simulink model "pi_SS_H2DF_2024a_GRU"  (R2024a)
settings: Solver=FixedStepAuto  StartTime=0.0  StopTime=inf  FixedStep=0.001  RelTol=1e-3  EnableMultiTasking=on
values from neighbouring files (symbols this model uses):
  C2C_NMPC = init_C2C_NMPC_H2DF(C2C_NMPC.expdata)    [run_SS_H2DF_control.m]
libraries: matrix_library x3, raspberrypiNetworklib x1
(part 3 of 3)

== system pi_SS_H2DF_2024a_GRU/main_C2C/post_processing/Subsystem1/Subsystem ==
  In1 : Inport
  In2 : Inport  Port=2
  In3 : Inport  Port=3
  In4 : Inport  Port=4
  " denormalizing reference1" : Subsystem
  " denormalizing reference2" : Subsystem
  " denormalizing reference3" : Subsystem
  " denormalizing reference4" : Subsystem
  Demux{,1..3} (4 alike) : Demux
  Mux{,1..3} (4 alike) : Mux
  Node_0 : Outport
  Node_1 : Outport  Port=2
  Node_2 : Outport  Port=3
  Node_3 : Outport  Port=4
  wires:
  Demux/1 -> " denormalizing reference1"/1(IMEP_norm)
  Demux/2 -> " denormalizing reference1"/2(NOX_norm)
  Demux/3 -> " denormalizing reference1"/3(soot_norm)
  Demux/4 -> " denormalizing reference1"/4(MPRR_norm)
  In1/1 -> Demux/1
  " denormalizing reference1"/1(IMEP) -> Mux/1
  " denormalizing reference1"/2(NOX) -> Mux/2
  " denormalizing reference1"/3(soot) -> Mux/3
  " denormalizing reference1"/4(MPRR) -> Mux/4
  " denormalizing reference2"/3(soot) -> Mux1/3
  Demux1/3 -> " denormalizing reference2"/3(soot_norm)
  In2/1 -> Demux1/1
  " denormalizing reference2"/2(NOX) -> Mux1/2
  " denormalizing reference2"/1(IMEP) -> Mux1/1
  Demux1/1 -> " denormalizing reference2"/1(IMEP_norm)
  Demux1/4 -> " denormalizing reference2"/4(MPRR_norm)
  Demux1/2 -> " denormalizing reference2"/2(NOX_norm)
  " denormalizing reference2"/4(MPRR) -> Mux1/4
  " denormalizing reference3"/3(soot) -> Mux2/3
  Demux2/3 -> " denormalizing reference3"/3(soot_norm)
  In3/1 -> Demux2/1
  " denormalizing reference3"/2(NOX) -> Mux2/2
  " denormalizing reference3"/1(IMEP) -> Mux2/1
  Demux2/1 -> " denormalizing reference3"/1(IMEP_norm)
  Demux2/4 -> " denormalizing reference3"/4(MPRR_norm)
  Demux2/2 -> " denormalizing reference3"/2(NOX_norm)
  " denormalizing reference3"/4(MPRR) -> Mux2/4
  " denormalizing reference4"/3(soot) -> Mux3/3
  Demux3/3 -> " denormalizing reference4"/3(soot_norm)
  In4/1 -> Demux3/1
  " denormalizing reference4"/2(NOX) -> Mux3/2
  " denormalizing reference4"/1(IMEP) -> Mux3/1
  Demux3/1 -> " denormalizing reference4"/1(IMEP_norm)
  Demux3/4 -> " denormalizing reference4"/4(MPRR_norm)
  Demux3/2 -> " denormalizing reference4"/2(NOX_norm)
  " denormalizing reference4"/4(MPRR) -> Mux3/4
  Mux/1 -> Node_0/1
  Mux1/1 -> Node_1/1
  Mux2/1 -> Node_2/1
  Mux3/1 -> Node_3/1

== system pi_SS_H2DF_2024a_GRU/main_C2C/post_processing/Subsystem1/Subsystem/ denormalizing reference1 ==
  IMEP_norm : Inport
  NOX_norm : Inport  Port=2
  soot_norm : Inport  Port=3
  MPRR_norm : Inport  Port=4
  Constant : Constant  Value=C2C_NMPC.Normalization.outputs.mean(1)
  Constant1 : Constant  Value=C2C_NMPC.Normalization.outputs.mean(2)
  Constant2 : Constant  Value=C2C_NMPC.Normalization.outputs.mean(3)
  Constant3 : Constant  Value=C2C_NMPC.Normalization.outputs.mean(4)
  Gain : Gain  Gain=C2C_NMPC.Normalization.outputs.std(1)
  Gain1 : Gain  Gain=C2C_NMPC.Normalization.outputs.std(2)
  Gain2 : Gain  Gain=C2C_NMPC.Normalization.outputs.std(3)
  Gain3 : Gain  Gain=C2C_NMPC.Normalization.outputs.std(4)
  Sum{1..3,5} (4 alike) : Sum  Inputs=|++
  IMEP : Outport
  NOX : Outport  Port=2
  soot : Outport  Port=3
  MPRR : Outport  Port=4
  wires:
  Gain/1 -> Sum5/1
  IMEP_norm/1 -> Gain/1
  Constant/1 -> Sum5/2
  Sum5/1 -> IMEP/1
  Gain1/1 -> Sum1/1
  Constant1/1 -> Sum1/2
  NOX_norm/1 -> Gain1/1
  Sum1/1 -> NOX/1
  Gain2/1 -> Sum2/1
  Constant2/1 -> Sum2/2
  soot_norm/1 -> Gain2/1
  Sum2/1 -> soot/1
  Gain3/1 -> Sum3/1
  Constant3/1 -> Sum3/2
  MPRR_norm/1 -> Gain3/1
  Sum3/1 -> MPRR/1

== system pi_SS_H2DF_2024a_GRU/main_C2C/post_processing/Subsystem1/Subsystem/ denormalizing reference2 ==
  IMEP_norm : Inport
  NOX_norm : Inport  Port=2
  soot_norm : Inport  Port=3
  MPRR_norm : Inport  Port=4
  Constant : Constant  Value=C2C_NMPC.Normalization.outputs.mean(1)
  Constant1 : Constant  Value=C2C_NMPC.Normalization.outputs.mean(2)
  Constant2 : Constant  Value=C2C_NMPC.Normalization.outputs.mean(3)
  Constant3 : Constant  Value=C2C_NMPC.Normalization.outputs.mean(4)
  Gain : Gain  Gain=C2C_NMPC.Normalization.outputs.std(1)
  Gain1 : Gain  Gain=C2C_NMPC.Normalization.outputs.std(2)
  Gain2 : Gain  Gain=C2C_NMPC.Normalization.outputs.std(3)
  Gain3 : Gain  Gain=C2C_NMPC.Normalization.outputs.std(4)
  Sum{1..3,5} (4 alike) : Sum  Inputs=|++
  IMEP : Outport
  NOX : Outport  Port=2
  soot : Outport  Port=3
  MPRR : Outport  Port=4
  wires:
  Gain/1 -> Sum5/1
  IMEP_norm/1 -> Gain/1
  Constant/1 -> Sum5/2
  Sum5/1 -> IMEP/1
  Gain1/1 -> Sum1/1
  Constant1/1 -> Sum1/2
  NOX_norm/1 -> Gain1/1
  Sum1/1 -> NOX/1
  Gain2/1 -> Sum2/1
  Constant2/1 -> Sum2/2
  soot_norm/1 -> Gain2/1
  Sum2/1 -> soot/1
  Gain3/1 -> Sum3/1
  Constant3/1 -> Sum3/2
  MPRR_norm/1 -> Gain3/1
  Sum3/1 -> MPRR/1

== system pi_SS_H2DF_2024a_GRU/main_C2C/post_processing/Subsystem1/Subsystem/ denormalizing reference3 ==
  IMEP_norm : Inport
  NOX_norm : Inport  Port=2
  soot_norm : Inport  Port=3
  MPRR_norm : Inport  Port=4
  Constant : Constant  Value=C2C_NMPC.Normalization.outputs.mean(1)
  Constant1 : Constant  Value=C2C_NMPC.Normalization.outputs.mean(2)
  Constant2 : Constant  Value=C2C_NMPC.Normalization.outputs.mean(3)
  Constant3 : Constant  Value=C2C_NMPC.Normalization.outputs.mean(4)
  Gain : Gain  Gain=C2C_NMPC.Normalization.outputs.std(1)
  Gain1 : Gain  Gain=C2C_NMPC.Normalization.outputs.std(2)
  Gain2 : Gain  Gain=C2C_NMPC.Normalization.outputs.std(3)
  Gain3 : Gain  Gain=C2C_NMPC.Normalization.outputs.std(4)
  Sum{1..3,5} (4 alike) : Sum  Inputs=|++
  IMEP : Outport
  NOX : Outport  Port=2
  soot : Outport  Port=3
  MPRR : Outport  Port=4
  wires:
  Gain/1 -> Sum5/1
  IMEP_norm/1 -> Gain/1
  Constant/1 -> Sum5/2
  Sum5/1 -> IMEP/1
  Gain1/1 -> Sum1/1
  Constant1/1 -> Sum1/2
  NOX_norm/1 -> Gain1/1
  Sum1/1 -> NOX/1
  Gain2/1 -> Sum2/1
  Constant2/1 -> Sum2/2
  soot_norm/1 -> Gain2/1
  Sum2/1 -> soot/1
  Gain3/1 -> Sum3/1
  Constant3/1 -> Sum3/2
  MPRR_norm/1 -> Gain3/1
  Sum3/1 -> MPRR/1

== system pi_SS_H2DF_2024a_GRU/main_C2C/post_processing/Subsystem1/Subsystem/ denormalizing reference4 ==
  IMEP_norm : Inport
  NOX_norm : Inport  Port=2
  soot_norm : Inport  Port=3
  MPRR_norm : Inport  Port=4
  Constant : Constant  Value=C2C_NMPC.Normalization.outputs.mean(1)
  Constant1 : Constant  Value=C2C_NMPC.Normalization.outputs.mean(2)
  Constant2 : Constant  Value=C2C_NMPC.Normalization.outputs.mean(3)
  Constant3 : Constant  Value=C2C_NMPC.Normalization.outputs.mean(4)
  Gain : Gain  Gain=C2C_NMPC.Normalization.outputs.std(1)
  Gain1 : Gain  Gain=C2C_NMPC.Normalization.outputs.std(2)
  Gain2 : Gain  Gain=C2C_NMPC.Normalization.outputs.std(3)
  Gain3 : Gain  Gain=C2C_NMPC.Normalization.outputs.std(4)
  Sum{1..3,5} (4 alike) : Sum  Inputs=|++
  IMEP : Outport
  NOX : Outport  Port=2
  soot : Outport  Port=3
  MPRR : Outport  Port=4
  wires:
  Gain/1 -> Sum5/1
  IMEP_norm/1 -> Gain/1
  Constant/1 -> Sum5/2
  Sum5/1 -> IMEP/1
  Gain1/1 -> Sum1/1
  Constant1/1 -> Sum1/2
  NOX_norm/1 -> Gain1/1
  Sum1/1 -> NOX/1
  Gain2/1 -> Sum2/1
  Constant2/1 -> Sum2/2
  soot_norm/1 -> Gain2/1
  Sum2/1 -> soot/1
  Gain3/1 -> Sum3/1
  Constant3/1 -> Sum3/2
  MPRR_norm/1 -> Gain3/1
  Sum3/1 -> MPRR/1

== matlab function pi_SS_H2DF_2024a_GRU/main_C2C/C2C_NMPC_n3/constraints1 soft /MATLAB Function2 ==
  data: value input; vector output; length input; init_vector input
function vector = fcn(value, length, init_vector)
init_vector(1:(size(value,1)*length)) = repmat(value, length, 1);
vector = init_vector;

== matlab function pi_SS_H2DF_2024a_GRU/main_C2C/C2C_NMPC_n3/constraints1 soft /MATLAB Function3 ==
  data: value input; vector output; length input; init_vector input
function vector = fcn(value, length, init_vector)
init_vector(1:(size(value,1)*length)) = repmat(value, length, 1);
vector = init_vector;

== matlab function pi_SS_H2DF_2024a_GRU/main_C2C/C2C_NMPC_n3/constraints1 soft /MATLAB Function4 ==
  data: value input; vector output; length input; init_vector input
function vector = fcn(value, length, init_vector)
init_vector(1:(size(value,1)*length)) = repmat(value, length, 1);
vector = init_vector;

== matlab function pi_SS_H2DF_2024a_GRU/main_C2C/C2C_NMPC_n3/constraints1 soft /MATLAB Function5 ==
  data: value input; vector output; length input; init_vector input
function vector = fcn(value, length, init_vector)
init_vector(1:(size(value,1)*length)) = repmat(value, length, 1);
vector = init_vector;

== matlab function pi_SS_H2DF_2024a_GRU/main_C2C/C2C_NMPC_n3/cost_function_weights/blkdiag Function ==
  data: u1 input; y output; u2 input; u3 input
 function y = fcn(u1,u2,u3)
y = reshape(blkdiag(u1, u2, u3),[],1);

== matlab function pi_SS_H2DF_2024a_GRU/main_C2C/C2C_NMPC_n3/cost_function_weights/blkdiag Function1 ==
  data: u1 input; y output; u2 input
function y = fcn(u1,u2)
y = reshape(blkdiag(u1, u2),[],1);

== matlab function pi_SS_H2DF_2024a_GRU/main_C2C/Subsystem/dyn_H2DF_state_augmentation/dyn_H2DF_state_augmentation ==
  data: last_LSTM_states input size=C2C_NMPC.Dims.n_cell_states+C2C_NMPC.Dims.n_hidden_states; LSTM_states output size=C2C_NMPC.Dims.n_cell_states+C2C_NMPC.Dims.n_hidden_states; controls input size=C2C_NMPC.Dims.n_controls; last_outputs_MC input size=C2C_NMPC.Dims.n_outputs; H2DF_Par parameter
 function LSTM_states = dyn_H2DF_state_augmentation_GRU(last_LSTM_states, controls, last_outputs_MC, H2DF_Par)

LSTM_states = dyn_H2DF_state_augmentation_GRU(last_LSTM_states,[controls; last_outputs_MC(1)], H2DF_Par);

== matlab function pi_SS_H2DF_2024a_GRU/main_C2C/C2C_NMPC_n3/constraints no soft/MATLAB Function ==
  data: value input; vector output; length input; init_vector input
function vector = fcn(value, length, init_vector)
init_vector(1:(size(value,1)*length)) = repmat(value, length, 1);
vector = init_vector;

== matlab function pi_SS_H2DF_2024a_GRU/main_C2C/C2C_NMPC_n3/constraints no soft/MATLAB Function1 ==
  data: value input; vector output; length input; init_vector input
function vector = fcn(value, length, init_vector)
init_vector(1:(size(value,1)*length)) = repmat(value, length, 1);
vector = init_vector;

== matlab function pi_SS_H2DF_2024a_GRU/main_C2C/C2C_NMPC_n3/constraints no soft/MATLAB Function2 ==
  data: value input; vector output; length input; init_vector input
function vector = fcn(value, length, init_vector)
init_vector(1:(size(value,1)*length)) = repmat(value, length, 1);
vector = init_vector;

== stateflow chart pi_SS_H2DF_2024a_GRU/Chart1 ==
  state wait
  (default) -> wait
  wait -> (junction 9) : [size>0]{call_main_C2C; call_tx_C2C}
  (junction 10) -> wait
  (junction 9) -> (junction 10)
  data: size input
  events: call_tx_C2C output FUNCTION_CALL_EVENT; call_main_C2C output FUNCTION_CALL_EVENT

== matlab function pi_SS_H2DF_2024a_GRU/main_C2C/C2C_NMPC_n3/constraints no soft/MATLAB Function3 ==
  data: value input; vector output; length input; init_vector input
function vector = fcn(value, length, init_vector)
init_vector(1:(size(value,1)*length)) = repmat(value, length, 1);
vector = init_vector;

== matlab function pi_SS_H2DF_2024a_GRU/main_C2C/C2C_NMPC_n3/constraints no soft/MATLAB Function4 ==
  data: value input; vector output; length input; init_vector input
function vector = fcn(value, length, init_vector)
init_vector(1:(size(value,1)*length)) = repmat(value, length, 1);
vector = init_vector;

== matlab function pi_SS_H2DF_2024a_GRU/main_C2C/C2C_NMPC_n3/constraints no soft/MATLAB Function5 ==
  data: value input; vector output; length input; init_vector input
function vector = fcn(value, length, init_vector)
init_vector(1:(size(value,1)*length)) = repmat(value, length, 1);
vector = init_vector;

== matlab function pi_SS_H2DF_2024a_GRU/main_C2C/C2C_NMPC_n3/constraints1 soft /MATLAB Function ==
  data: value input; vector output; length input; init_vector input
function vector = fcn(value, length, init_vector)
init_vector(1:(size(value,1)*length)) = repmat(value, length, 1);
vector = init_vector;

== matlab function pi_SS_H2DF_2024a_GRU/main_C2C/C2C_NMPC_n3/constraints1 soft /MATLAB Function1 ==
  data: value input; vector output; length input; init_vector input
function vector = fcn(value, length, init_vector)
init_vector(1:(size(value,1)*length)) = repmat(value, length, 1);
vector = init_vector;
